simulink model "validation_simulations_elena"  (R2019b)
settings: Solver=FixedStepAuto  StartTime=0.0  StopTime=20  FixedStep=0.002  RelTol=1e-3
undefined symbols (not defined in the file or in its folder): Ao, Bo, Co, kalmf, Klqi_int, Klqi_state, Kpp_int, Kpp_state, Parameters
settings Model: Creator=Samsung  LastModifiedBy=Samsung

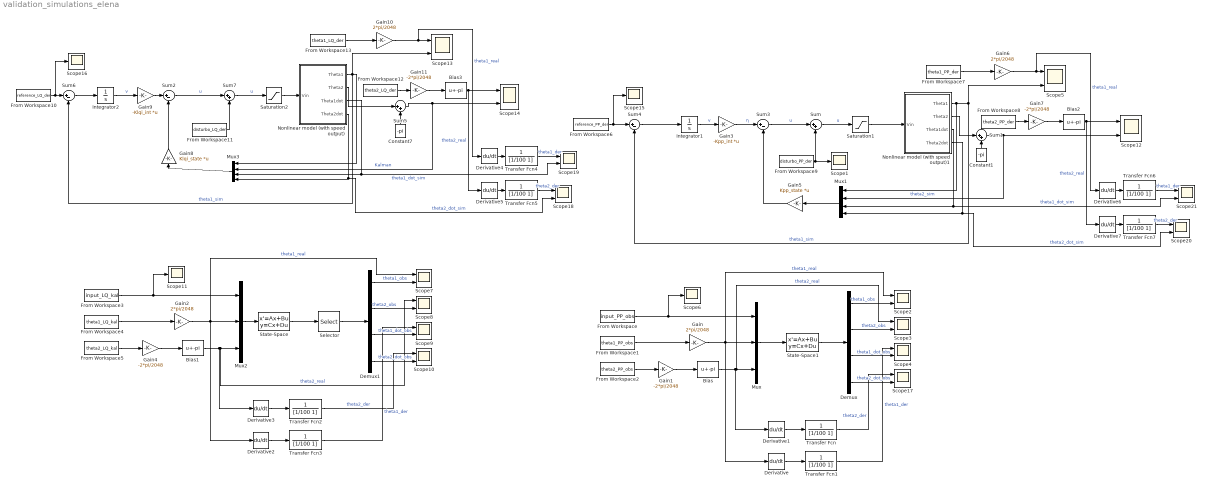
== system validation_simulations_elena ==
  Bias{,1..3} (4 alike) : Bias  Bias=-pi
  Constant1 : Constant  Value=-pi
  Constant7 : Constant  Value=-pi
  Demux : Demux
  Demux1 : Demux
  Derivative{,1..7} (8 alike) : Derivative
  From Workspace : FromWorkspace  VariableName=input_PP_obs  SampleTime=0
  From Workspace1 : FromWorkspace  VariableName=theta1_PP_obs  SampleTime=0
  From Workspace10 : FromWorkspace  VariableName=reference_LQ_der  SampleTime=0
  From Workspace11 : FromWorkspace  VariableName=disturbo_LQ_der  SampleTime=0
  From Workspace12 : FromWorkspace  VariableName=theta2_LQ_der  SampleTime=0
  From Workspace13 : FromWorkspace  VariableName=theta1_LQ_der  SampleTime=0
  From Workspace2 : FromWorkspace  VariableName=theta2_PP_obs  SampleTime=0
  From Workspace3 : FromWorkspace  VariableName=input_LQ_kal  SampleTime=0
  From Workspace4 : FromWorkspace  VariableName=theta1_LQ_kal  SampleTime=0
  From Workspace5 : FromWorkspace  VariableName=theta2_LQ_kal  SampleTime=0
  From Workspace6 : FromWorkspace  VariableName=reference_PP_der  SampleTime=0
  From Workspace7 : FromWorkspace  VariableName=theta1_PP_der  SampleTime=0
  From Workspace8 : FromWorkspace  VariableName=theta2_PP_der  SampleTime=0
  From Workspace9 : FromWorkspace  VariableName=disturbo_PP_der  SampleTime=0
  Gain{,2,6,10} (4 alike) : Gain  Gain=2*pi/2048
  Gain{1,4,7,11} (4 alike) : Gain  Gain=-2*pi/2048
  Gain3 : Gain  Gain=-Kpp_int  Multiplication=Matrix(K*u)
  Gain5 : Gain  Gain=Kpp_state  Multiplication=Matrix(K*u)
  Gain8 : Gain  Gain=Klqi_state  Multiplication=Matrix(K*u)
  Gain9 : Gain  Gain=-Klqi_int  Multiplication=Matrix(K*u)
  Integrator1 : Integrator
  Integrator2 : Integrator
  Mux : Mux  Inputs=3
  Mux1 : Mux
  Mux2 : Mux  Inputs=3
  Mux3 : Mux
  Nonlinear model (with speed output) : Subsystem
  Nonlinear model (with speed output)1 : Subsystem
  Saturation1 : Saturate  UpperLimit=10  LowerLimit=-10
  Saturation2 : Saturate  UpperLimit=10  LowerLimit=-10
  Scope{1,6,11,15..16} (5 alike) : Scope
  Scope{2..5,7..10,12..14,17..21} (16 alike) : Scope  NumInputPorts=2
  Selector : Selector  InputPortWidth=6  IndexOptions=Index vector (dialog)  Indices=[3,4,5,6]  OutputSizes=1
  State-Space : StateSpace  A=kalmf.A  B=kalmf.B  C=kalmf.C  D=kalmf.D  InitialCondition=[0,0,0,0]
  State-Space1 : StateSpace  A=Ao  B=Bo  C=Co  D=zeros(4,3)  InitialCondition=[0,0,0,0]
  Sum{,1,5,7} (4 alike) : Sum  Inputs=|++
  Sum{2..4,6} (4 alike) : Sum  Inputs=|+-
  Transfer Fcn{,1..7} (8 alike) : TransferFcn  Denominator=[1/100 1]
  wires:
  Mux1/1 -> Gain5/1
  Sum4/1 -> Integrator1/1
  Nonlinear model (with speed output)1/2(Theta2) -> Sum1/1
  Gain5/1 -> Sum3/2
  Nonlinear model (with speed output)1/1(Theta1) -> Mux1/1, Scope5/2, Sum4/2  "theta1_sim"
  Sum/1 -> Saturation1/1  "u"
  Constant1/1 -> Sum1/2
  Saturation1/1 -> Nonlinear model (with speed output)1/1(Vin)
  Integrator1/1 -> Gain3/1  "v"
  Gain3/1 -> Sum3/1  "η"
  Sum1/1 -> Scope12/2, Mux1/2  "theta2_sim"
  Mux/1 -> State-Space1/1
  State-Space1/1 -> Demux/1
  Gain/1 -> Scope2/1, Derivative/1, Mux/2  "theta1_real"
  Gain1/1 -> Bias/1
  Demux/1 -> Scope2/2  "theta1_obs"
  Demux/2 -> Scope3/2  "theta2_obs"
  Demux/3 -> Scope4/2  "theta1_dot_obs"
  Demux/4 -> Scope17/2  "theta2_dot_obs"
  Derivative1/1 -> Transfer Fcn/1
  Derivative/1 -> Transfer Fcn1/1
  Transfer Fcn/1 -> Scope17/1  "theta2_der"
  Transfer Fcn1/1 -> Scope4/1  "theta1_der"
  From Workspace1/1 -> Gain/1
  From Workspace2/1 -> Gain1/1
  From Workspace/1 -> Scope6/1, Mux/1
  Bias/1 -> Scope3/1, Mux/3, Derivative1/1  "theta2_real"
  State-Space/1 -> Selector/1
  Mux2/1 -> State-Space/1
  From Workspace5/1 -> Gain4/1
  Transfer Fcn2/1 -> Scope10/1  "theta2_der"
  Demux1/1 -> Scope7/2  "theta1_obs"
  Bias1/1 -> Scope8/1, Mux2/3, Derivative3/1  "theta2_real"
  From Workspace3/1 -> Scope11/1, Mux2/1
  Demux1/2 -> Scope8/2  "theta2_obs"
  From Workspace4/1 -> Gain2/1
  Transfer Fcn3/1 -> Scope9/1  "theta1_der"
  Gain2/1 -> Scope7/1, Derivative2/1, Mux2/2  "theta1_real"
  Demux1/4 -> Scope10/2  "theta2_dot_obs"
  Gain4/1 -> Bias1/1
  Demux1/3 -> Scope9/2  "theta1_dot_obs"
  Derivative3/1 -> Transfer Fcn2/1
  Derivative2/1 -> Transfer Fcn3/1
  Selector/1 -> Demux1/1
  From Workspace6/1 -> Scope15/1, Sum4/1
  From Workspace7/1 -> Gain6/1
  From Workspace8/1 -> Gain7/1
  Gain7/1 -> Bias2/1
  Sum3/1 -> Sum/1  "u"
  From Workspace9/1 -> Sum/2, Scope1/1
  Sum7/1 -> Saturation2/1  "u"
  Saturation2/1 -> Nonlinear model (with speed output)/1(Vin)
  Nonlinear model (with speed output)/2(Theta2) -> Sum5/1
  Gain9/1 -> Sum2/1
  Constant7/1 -> Sum5/2
  Mux3/1 -> Gain8/1
  Integrator2/1 -> Gain9/1  "v"
  Gain8/1 -> Sum2/2
  Sum6/1 -> Integrator2/1
  Sum5/1 -> Scope14/2, Mux3/2  "Kalman"
  From Workspace10/1 -> Scope16/1, Sum6/1
  Sum2/1 -> Sum7/1  "u"
  From Workspace11/1 -> Sum7/2
  From Workspace12/1 -> Gain11/1
  From Workspace13/1 -> Gain10/1
  Bias3/1 -> Derivative5/1, Scope14/1  "theta2_real"
  Nonlinear model (with speed output)/1(Theta1) -> Scope13/2, Mux3/1, Sum6/2  "theta1_sim"
  Gain10/1 -> Scope13/1, Derivative4/1  "theta1_real"
  Gain11/1 -> Bias3/1
  Nonlinear model (with speed output)/3(Theta1dot) -> Scope19/2, Mux3/3  "theta1_dot_sim"
  Nonlinear model (with speed output)/4(Theta2dot) -> Scope18/2, Mux3/4  "theta2_dot_sim"
  Derivative4/1 -> Transfer Fcn4/1
  Derivative5/1 -> Transfer Fcn5/1
  Transfer Fcn5/1 -> Scope18/1  "theta2_der"
  Transfer Fcn4/1 -> Scope19/1  "theta1_der"
  Bias2/1 -> Derivative7/1, Scope12/1  "theta2_real"
  Derivative6/1 -> Transfer Fcn6/1
  Derivative7/1 -> Transfer Fcn7/1
  Gain6/1 -> Scope5/1, Derivative6/1  "theta1_real"
  Transfer Fcn7/1 -> Scope20/1  "theta2_der"
  Transfer Fcn6/1 -> Scope21/1  "theta1_der"
  Nonlinear model (with speed output)1/4(Theta2dot) -> Mux1/4, Scope20/2  "theta2_dot_sim"
  Nonlinear model (with speed output)1/3(Theta1dot) -> Mux1/3, Scope21/2  "theta1_dot_sim"

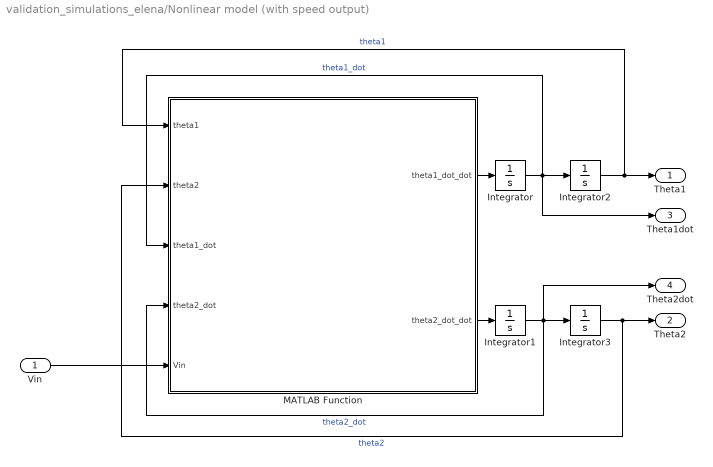
== system validation_simulations_elena/Nonlinear model (with speed output) ==
  Vin : Inport
  Integrator : Integrator
  Integrator1 : Integrator
  Integrator2 : Integrator
  Integrator3 : Integrator  InitialCondition=pi
  MATLAB Function : MATLAB Function  TreatAsAtomicUnit=on  mask{Pars=Parameters}
      mask prompts: Pars "Struct containing model parameters"
  Theta1 : Outport
  Theta2 : Outport  Port=2
  Theta1dot : Outport  Port=3
  Theta2dot : Outport  Port=4
  wires:
  Integrator/1 -> Theta1dot/1, MATLAB Function/3(theta1_dot), Integrator2/1  "theta1_dot"
  Integrator1/1 -> Theta2dot/1, MATLAB Function/4(theta2_dot), Integrator3/1  "theta2_dot"
  MATLAB Function/1(theta1_dot_dot) -> Integrator/1
  Integrator3/1 -> Theta2/1, MATLAB Function/2(theta2)  "theta2"
  MATLAB Function/2(theta2_dot_dot) -> Integrator1/1
  Integrator2/1 -> MATLAB Function/1(theta1), Theta1/1  "theta1"
  Vin/1 -> MATLAB Function/5(Vin)

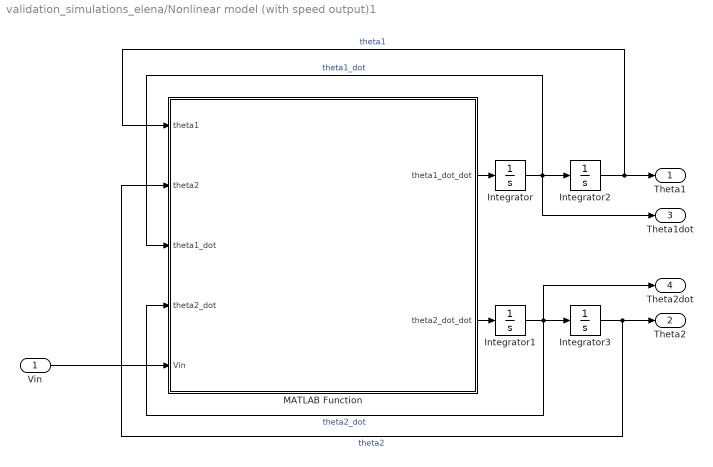
== system validation_simulations_elena/Nonlinear model (with speed output)1 ==
  Vin : Inport
  Integrator : Integrator
  Integrator1 : Integrator
  Integrator2 : Integrator  InitialCondition=0.1
  Integrator3 : Integrator  InitialCondition=pi+0.04
  MATLAB Function : MATLAB Function  TreatAsAtomicUnit=on  mask{Pars=Parameters}
      mask prompts: Pars "Struct containing model parameters"
  Theta1 : Outport
  Theta2 : Outport  Port=2
  Theta1dot : Outport  Port=3
  Theta2dot : Outport  Port=4
  wires:
  Integrator/1 -> Theta1dot/1, MATLAB Function/3(theta1_dot), Integrator2/1  "theta1_dot"
  Integrator1/1 -> Theta2dot/1, MATLAB Function/4(theta2_dot), Integrator3/1  "theta2_dot"
  MATLAB Function/1(theta1_dot_dot) -> Integrator/1
  Integrator3/1 -> Theta2/1, MATLAB Function/2(theta2)  "theta2"
  MATLAB Function/2(theta2_dot_dot) -> Integrator1/1
  Integrator2/1 -> MATLAB Function/1(theta1), Theta1/1  "theta1"
  Vin/1 -> MATLAB Function/5(Vin)

== matlab function validation_simulations_elena/Nonlinear model (with speed output)/MATLAB Function ==
  data: theta1 input; theta1_dot_dot output; theta2 input; theta1_dot input; theta2_dot input; Vin input; theta2_dot_dot output; Pars parameter
function [theta1_dot_dot,theta2_dot_dot] = fcn(theta1, theta2, theta1_dot, theta2_dot,Vin, Pars)

   k1 = Pars.Jeq + Pars.m2*(Pars.l1^2 + Pars.x2^2*sin(theta2)^2);
   k2 = Pars.m2*Pars.l1*Pars.x2*cos(theta2);
   k3 = 2*Pars.m2*Pars.x2^2*sin(theta2)*cos(theta2)*theta1_dot*theta2_dot - Pars.m2*Pars.l1*Pars.x2*sin(theta2)*theta2_dot^2 +Pars.Ks*theta1 - Pars.Km/Pars.Rm*Vin + (Pars.Km^2)/Pars.Rm*theta1_dot + Pars.Kf1*theta1_dot;
   k4 = Pars.m2*Pars.l1*Pars.x2*cos(theta2);
   k5 = Pars.m2*Pars.x2^2 + Pars.I2;
   k6 = - Pars.m2*Pars.x2^2*sin(theta2)*cos(theta2)*theta1_dot^2 + Pars.m2*Pars.g*Pars.x2*sin(theta2) + Pars.Kf2*theta2_dot;


theta1_dot_dot = (k2*k6 - k3*k5)/(k1*k5 - k2*k4);
theta2_dot_dot = -(k1*k6 - k3*k4)/(k1*k5 - k2*k4);

== matlab function validation_simulations_elena/Nonlinear model (with speed output)1/MATLAB Function ==
  data: theta1 input; theta1_dot_dot output; theta2 input; theta1_dot input; theta2_dot input; Vin input; theta2_dot_dot output; Pars parameter
function [theta1_dot_dot,theta2_dot_dot] = fcn(theta1, theta2, theta1_dot, theta2_dot,Vin, Pars)

   k1 = Pars.Jeq + Pars.m2*(Pars.l1^2 + Pars.x2^2*sin(theta2)^2);
   k2 = Pars.m2*Pars.l1*Pars.x2*cos(theta2);
   k3 = 2*Pars.m2*Pars.x2^2*sin(theta2)*cos(theta2)*theta1_dot*theta2_dot - Pars.m2*Pars.l1*Pars.x2*sin(theta2)*theta2_dot^2 +Pars.Ks*theta1 - Pars.Km/Pars.Rm*Vin + (Pars.Km^2)/Pars.Rm*theta1_dot + Pars.Kf1*theta1_dot;
   k4 = Pars.m2*Pars.l1*Pars.x2*cos(theta2);
   k5 = Pars.m2*Pars.x2^2 + Pars.I2;
   k6 = - Pars.m2*Pars.x2^2*sin(theta2)*cos(theta2)*theta1_dot^2 + Pars.m2*Pars.g*Pars.x2*sin(theta2) + Pars.Kf2*theta2_dot;


theta1_dot_dot = (k2*k6 - k3*k5)/(k1*k5 - k2*k4);
theta2_dot_dot = -(k1*k6 - k3*k4)/(k1*k5 - k2*k4);
